simulink model "Model_1"  (R2020b)
settings: Solver=VariableStepAuto  StartTime=0.0  StopTime=2000  RelTol=1e-3
settings Model: EnablePacing=on  PacingRate=50  Creator=samar  LastModifiedBy=samar

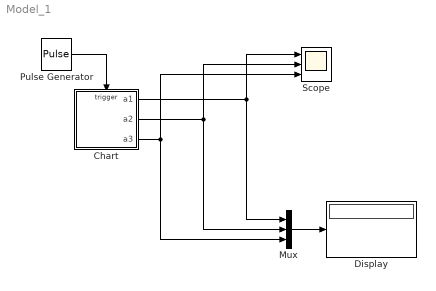
== system Model_1 ==
  Chart : Stateflow chart  TreatAsAtomicUnit=on
  Display : Display
  Mux : Mux  Inputs=3
  Pulse Generator : DiscretePulseGenerator  PulseType=Time based  Period=10  PulseWidth=5
  Scope : Scope  NumInputPorts=3
  wires:
  Pulse Generator/1 -> Chart/Trigger
  Chart/2(a2) -> Mux/2, Scope/2
  Chart/3(a3) -> Scope/3, Mux/3
  Mux/1 -> Display/1
  Chart/1(a1) -> Mux/1, Scope/1

== stateflow chart Model_1/Chart ==
  settings: executeAtInitialization=1
  state state1 [parallel]
    settings: executionOrder=1
    state two1
      en:
      a1=2;
    state three1
      en:
      a1=3;
    state one1
      en:
      a1=1;
    state four1
      en:
      a1=4;
    state zero1
      en:
      a1=0;
    one1 -> two1 : event1
    two1 -> three1 : event1
    zero1 -> one1 : event1
    three1 -> four1 : event1
    four1 -> zero1 : event1/{state2.event2}
    (default) -> zero1
  state state2 [parallel]
    settings: executionOrder=2
    state two2
      en:
      a2=2;
    state one2
      en:
      a2=1;
    state three2
      en:
      a2=3;
    state zero2
      en:
      a2=0;
    state four2
      en:
      a2=4;
    two2 -> three2 : event2
    one2 -> two2 : event2
    zero2 -> one2 : event2
    three2 -> four2 : event2
    (default) -> zero2
    four2 -> zero2 : event2/{state3.event3}
  state state3 [parallel]
    settings: executionOrder=3
    state two3
      en:
      a3=2;
    state one3
      en:
      a3=1;
    state three3
      en:
      a3=3;
    state four3
      en:
      a3=4;
    state zero3
      en:
      a3=0;
    one3 -> two3 : event3
    two3 -> three3 : event3
    zero3 -> one3 : event3
    three3 -> four3 : event3
    (default) -> zero3
    four3 -> zero3 : event3
  data: a1 output; a2 output; a3 output
  events: event2 local FUNCTION_CALL_EVENT; event3 local FUNCTION_CALL_EVENT; event1 input RISING_EDGE_EVENT
